simulink model "linearizacijaRezervoari"  (R2018a)
settings: Solver=VariableStepAuto  StartTime=0.0  StopTime=6500  RelTol=1e-3
values from neighbouring files (symbols this model uses):
  a = c/(pi*(h1^(3/2))*(2*R-h1))    [konstanteLinearizacija.m]
  A = [-a 0; a -a]    [konstanteLinearizacija.m]
  A0 = 0.01    [konstanteLinearizacija.m]
  A1 = pi*h1*(R-h1/2)    (= 1.50796447372)    [konstanteLinearizacija.m]
  b = 2/(pi*h1*(2*R-h1))    (= 0.663145596216)    [konstanteLinearizacija.m]
  B = [b; 0]    [konstanteLinearizacija.m]
  C = [0 1]    [konstanteLinearizacija.m]
  D = 0    [konstanteLinearizacija.m]
  g = 9.81    [konstanteLinearizacija.m]
  h2 = 0.8    [konstanteLinearizacija.m]
  q0 = c*sqrt(h1)    [konstanteLinearizacija.m]
  qu_max = 0.04    [konstanteLinearizacija.m]
  T = 1    [konstanteLinearizacija.m]
settings Model: Creator=Asus  LastModifiedBy=Asus

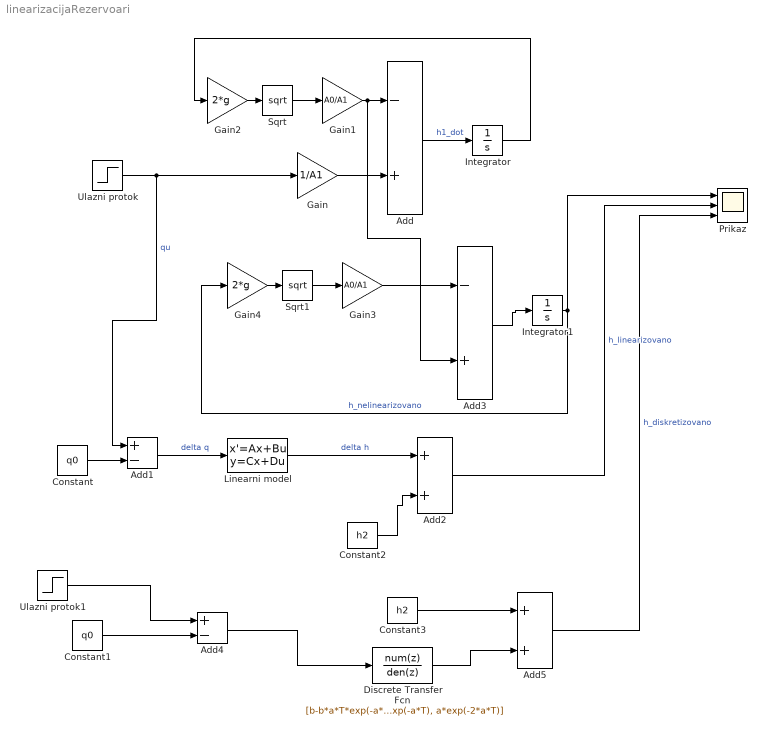
== system linearizacijaRezervoari ==
  Add : Sum  Inputs=-+
  Add1 : Sum  Inputs=+-
  Add2 : Sum
  Add3 : Sum  Inputs=-+
  Add4 : Sum  Inputs=+-
  Add5 : Sum
  Constant : Constant  Value=q0
  Constant1 : Constant  Value=q0  SampleTime=T
  Constant2 : Constant  Value=h2
  Constant3 : Constant  Value=h2  SampleTime=T
  Discrete Transfer Fcn : DiscreteTransferFcn  Numerator=[b-b*a*T*exp(-a*T)-b*exp(-a*T), b*exp(-2*a*T)-b*exp(-a*T)+b*a*T*exp(-a*T)]  Denominator=[a, -2*a*exp(-a*T), a*exp(-2*a*T)]
  Gain : Gain  Gain=1/A1
  Gain1 : Gain  Gain=A0/A1
  Gain2 : Gain  Gain=2*g
  Gain3 : Gain  Gain=A0/A1
  Gain4 : Gain  Gain=2*g
  Integrator : Integrator
  Integrator1 : Integrator
  Linearni model : StateSpace  A=A  B=B  C=C  D=D  InitialCondition=0
  Prikaz : Scope  NumInputPorts=3
  Sqrt : Sqrt  SaturateOnIntegerOverflow=on
  Sqrt1 : Sqrt  SaturateOnIntegerOverflow=on
  Ulazni protok : Step  Time=100  After=qu_max  SampleTime=0
  Ulazni protok1 : Step  Time=100  After=qu_max  SampleTime=T
  wires:
  Sqrt/1 -> Gain1/1
  Gain/1 -> Add/2
  Gain2/1 -> Sqrt/1
  Add/1 -> Integrator/1  "h1_dot"
  Integrator/1 -> Gain2/1
  Constant/1 -> Add1/2
  Ulazni protok/1 -> Add1/1, Gain/1  "qu"
  Add1/1 -> Linearni model/1  "delta q"
  Linearni model/1 -> Add2/1  "delta h"
  Add3/1 -> Integrator1/1
  Gain4/1 -> Sqrt1/1
  Sqrt1/1 -> Gain3/1
  Gain3/1 -> Add3/1
  Integrator1/1 -> Prikaz/1, Gain4/1  "h_nelinearizovano"
  Gain1/1 -> Add3/2, Add/1
  Add2/1 -> Prikaz/2  "h_linearizovano"
  Constant2/1 -> Add2/2
  Add4/1 -> Discrete Transfer Fcn/1
  Discrete Transfer Fcn/1 -> Add5/2
  Add5/1 -> Prikaz/3  "h_diskretizovano"
  Constant1/1 -> Add4/2
  Ulazni protok1/1 -> Add4/1
  Constant3/1 -> Add5/1
